simulink model "AMCLIB_SpeedLoop_BAM"  (Simulink 9.3)
settings: Solver=VariableStepAuto  StartTime=0.0  StopTime=10.0  RelTol=1e-3
settings Model: Creator=nxa18952  LastModifiedBy=nxa18952
settings DataIOCC: SaveFormat=Dataset  SignalLoggingSaveFormat=Dataset  ReturnWorkspaceOutputs=on
settings OptimizationCC: LifeSpan=auto
settings DebuggingCC: UnderspecifiedInitializationDetection=Simplified  MergeDetectMultiDrivingBlocksExec=error  FcnCallInpInsideContextMsg=error  SFUnexpectedBacktrackingDiag=error  SFNoUnconditionalDefaultTransitionDiag=error  SFExecutionAtInitializationDiag=warning  ArithmeticOperatorsInVariantConditions=error
settings HardwareCC: ProdBitPerPointer=64  ProdBitPerSizeT=64  ProdBitPerPtrDiffT=64  ProdLargestAtomicFloat=Float  ProdIntDivRoundTo=Zero  ProdEndianess=LittleEndian  ProdWordSize=64  ProdHWDeviceType=Intel->x86-64 (Windows64)
settings ModelReferenceCC: PropagateSignalLabelsOutOfModel=on
settings SFSimCC: SimUseLocalCustomCode=on
settings RTWCC: RTWUseLocalCustomCode=on
settings CodeAppCC: StateflowObjectComments=off
settings GRTTargetCC: TargetLangStandard=C99 (ISO)  CombineOutputUpdateFcns=on  GRTInterface=off
settings ConfigComp: CovMetricSettings=dwe  CovHtmlReporting=off  CovSaveCumulativeToWorkspaceVar=off  CovSaveSingleToWorkspaceVar=off  CovExternalEMLEnable=on

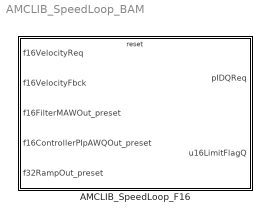
== system AMCLIB_SpeedLoop_BAM ==
  AMCLIB_SpeedLoop_F16 : Subsystem  TreatAsAtomicUnit=on  mask(AMCLIB_SpeedLoop_F16){showStates=Hide (faster execution), resetStatesEnable=Pre-set according to the first set of inputs after reset, showDebugOutputs=Hide, u16NSamplesW=0, f16PropGainQ=0, f16IntegGainQ=0, s16PropGainShiftQ=0, s16IntegGainShiftQ=0, f16LowerLimitQ=0, f16UpperLimitQ=0, f32RampUp=0, f32RampDown=0}
      mask prompts: showStates "Show internal states"; resetStatesEnable "Internal state after reset"; showDebugOutputs "Show debugging outputs"; u16NSamplesW "u16NSamplesW (GDFLIB_FilterMA - recalculated smoothing factor)"; f16PropGainQ "f16PropGainQ (GFLIB_ControllerPIpAW - proportional gain)"; f16IntegGainQ "f16IntegGainQ (GFLIB_ControllerPIpAW - integral gain)"; s16PropGainShiftQ "s16PropGainShiftQ (GFLIB_ControllerPIpAW - scaling bitwise shift applied to the proportional gain)"; s16IntegGainShiftQ "s16IntegGainShiftQ (GFLIB_ControllerPIpAW - scaling bitwise shift applied to the integral gain)"; f16LowerLimitQ "f16LowerLimitQ (GFLIB_ControllerPIpAW - lower limit)"; f16UpperLimitQ "f16UpperLimitQ (GFLIB_ControllerPIpAW - upper limit)"; f32RampUp "f32RampUp (Ramp up increment coefficient)"; f32RampDown "f32RampDown (Ramp decrement coefficient)"
      mask help: Speed loop controller for the PMSM field-oriented control algorithm in 16-bit fixed-point fractional implementation. This block supports re-initialization of the internal state during simulation. If the block is reset, the outputs of the MA filter, PI controller, and the ramp will be aligned with the inputs f16FilterMAWOut_preset, f16ControllerPIpAWQOut_preset, and f32RampOut_preset. Refer to the AMMCLIB User's Guide for further details.
      mask init:
      | if ~evalin('base','exist(''tS8'',''var'')')
      |   if (2 ~= exist('SWLIBS_Typedefs.mat','file'))
      |       error('File SWLIBS_Typedefs.mat is not on the Matlab path. Please add the AMMCLIB "bam" folder in the Matlab Search Path.');
      |   else
      |       evalin('base', 'load(''SWLIBS_Typedefs.mat'')');
      |   end
      | end
      | if showStates == 1
      |     % hidden state variables
      |     if strcmp(get_param([gcb '/u16NSamplesW'], 'BlockType'), 'Inport')
      |         posblk = get_param(gcb, 'Position');
      | 
      |         pos = get_param(    [gcb, '/u16NSamplesW'], 'Position');
      |         orient = get_param( [gcb, '/u16NSamplesW'], 'Orientation');
      |         delete_block(       [gcb, '/u16NSamplesW']);
      |         add_block('built-in/Ground', [gcb, '/u16NSamplesW'], 'Position', pos, 'Orientation', orient);
      | 
      |         pos = get_param(    [gcb, '/f16PropGainQ'], 'Position');
      |         orient = get_param( [gcb, '/f16PropGainQ'], 'Orientation');
      |         delete_block(       [gcb, '/f16PropGainQ']);
      |         add_block('built-in/Ground', [gcb, '/f16PropGainQ'], 'Position', pos, 'Orientation', orient);
      | 
      |         pos = get_param(    [gcb, '/f16IntegGainQ'], 'Position');
      |         orient = get_param( [gcb, '/f16IntegGainQ'], 'Orientation');
      |         delete_block(       [gcb, '/f16IntegGainQ']);
      |         add_block('built-in/Ground', [gcb, '/f16IntegGainQ'], 'Position', pos, 'Orientation', orient);
      | 
      |         pos = get_param(    [gcb, '/s16PropGainShiftQ'], 'Position');
      |         orient = get_param( [gcb, '/s16PropGainShiftQ'], 'Orientation');
      |         delete_block(       [gcb, '/s16PropGainShiftQ']);
      |         add_block('built-in/Ground', [gcb, '/s16PropGainShiftQ'], 'Position', pos, 'Orientation', orient);
      | 
      |         pos = get_param(    [gcb, '/s16IntegGainShiftQ'], 'Position');
      |         orient = get_param( [gcb, '/s16IntegGainShiftQ'], 'Orientation');
      |         delete_block(       [gcb, '/s16IntegGainShiftQ']);
      |         add_block('built-in/Ground', [gcb, '/s16IntegGainShiftQ'], 'Position', pos, 'Orientation', orient);
      | 
      |         pos = get_param(    [gcb, '/f16LowerLimitQ'], 'Position');
      |         orient = get_param( [gcb, '/f16LowerLimitQ'], 'Orientation');
      |         delete_block(       [gcb, '/f16LowerLimitQ']);
      |         add_block('built-in/Ground', [gcb, '/f16LowerLimitQ'], 'Position', pos, 'Orientation', orient);
      | 
      |         pos = get_param(    [gcb, '/f16UpperLimitQ'], 'Position');
      |         orient = get_param( [gcb, '/f16UpperLimitQ'], 'Orientation');
      |         delete_block(       [gcb, '/f16UpperLimitQ']);
      |         add_block('built-in/Ground', [gcb, '/f16UpperLimitQ'], 'Position', pos, 'Orientation', orient);
      | 
      |         pos = get_param(    [gcb, '/f32RampUp'], 'Position');
      |         orient = get_param( [gcb, '/f32RampUp'], 'Orientation');
      |         delete_block(       [gcb, '/f32RampUp']);
      |         add_block('built-in/Ground', [gcb, '/f32RampUp'], 'Position', pos, 'Orientation', orient);
      | 
      |         pos = get_param(    [gcb, '/f32RampDown'], 'Position');
      |         orient = get_param( [gcb, '/f32RampDown'], 'Orientation');
      |         delete_block(       [gcb, '/f32RampDown']);
      |         add_block('built-in/Ground', [gcb, '/f32RampDown'], 'Position', pos, 'Orientation', orient);
      | 
      |         pos = get_param(    [gcb, '/f32AccW'], 'Position');
      |         orient = get_param( [gcb, '/f32AccW'], 'Orientation');
      |         delete_block(       [gcb, '/f32AccW']);
      |         add_block('built-in/Ground', [gcb, '/f32AccW'], 'Position', pos, 'Orientation', orient);
      | 
      |         pos = get_param(    [gcb, '/f32IntegPartK_1Q'], 'Position');
      |         orient = get_param( [gcb, '/f32IntegPartK_1Q'], 'Orientation');
      |         delete_block(       [gcb, '/f32IntegPartK_1Q']);
      |         add_block('built-in/Ground', [gcb, '/f32IntegPartK_1Q'], 'Position', pos, 'Orientation', orient);
      | 
      |         pos = get_param(    [gcb, '/f16InK_1Q'], 'Position');
      |         orient = get_param( [gcb, '/f16InK_1Q'], 'Orientation');
      |         delete_block(       [gcb, '/f16InK_1Q']);
      |         add_block('built-in/Ground', [gcb, '/f16InK_1Q'], 'Position', pos, 'Orientation', orient);
      | 
      |         pos = get_param(    [gcb, '/f32State'], 'Position');
      |         orient = get_param( [gcb, '/f32State'], 'Orientation');
      |         delete_block(       [gcb, '/f32State']);
      |         add_block('built-in/Ground', [gcb, '/f32State'], 'Position', pos, 'Orientation', orient);
      | 
      | 
      |         pos = get_param(    [gcb '/f32AccW_Out'], 'Position');
      |         orient = get_param( [gcb '/f32AccW_Out'], 'Orientation');
      |         delete_block(       [gcb '/f32AccW_Out']);
      |         add_block('built-in/Terminator', [gcb '/f32AccW_Out'], 'Position', pos, 'Orientation', orient);
      | 
      |         pos = get_param(    [gcb '/f32IntegPartK_1Q_Out'], 'Position');
      |         orient = get_param( [gcb '/f32IntegPartK_1Q_Out'], 'Orientation');
      |         delete_block(       [gcb '/f32IntegPartK_1Q_Out']);
      |         add_block('built-in/Terminator', [gcb '/f32IntegPartK_1Q_Out'], 'Position', pos, 'Orientation', orient);
      | 
      |         pos = get_param(    [gcb '/f16InK_1Q_Out'], 'Position');
      |         orient = get_param( [gcb '/f16InK_1Q_Out'], 'Orientation');
      |         delete_block(       [gcb '/f16InK_1Q_Out']);
      |         add_block('built-in/Terminator', [gcb '/f16InK_1Q_Out'], 'Position', pos, 'Orientation', orient);
      | 
      |         pos = get_param(    [gcb '/f32State_Out'], 'Position');
      |         orient = get_param( [gcb '/f32State_Out'], 'Orientation');
      |         delete_block(       [gcb '/f32State_Out']);
      |         add_block('built-in/Terminator', [gcb '/f32State_Out'], 'Position', pos, 'Orientation', orient);
      | 
      | 
      |         if strcmp(get_param([gcb '/f16WReqFilt'], 'BlockType'), 'Outport')
      |             pos = get_param(    [gcb '/f16WReqFilt'], 'Position');
      |             orient = get_param( [gcb '/f16WReqFilt'], 'Orientation');
      |             delete_block(       [gcb '/f16WReqFilt']);
      |             add_block('built-in/Terminator', [gcb '/f16WReqFilt'], 'Position', pos, 'Orientation', orient);
      | 
      |             pos = get_param(    [gcb '/f16WErr'], 'Position');
      |             orient = get_param( [gcb '/f16WErr'], 'Orientation');
      |             delete_block(       [gcb '/f16WErr']);
      |             add_block('built-in/Terminator', [gcb '/f16WErr'], 'Position', pos, 'Orientation', orient);
      | 
      |             pos = get_param(    [gcb '/f16WFbckFilt'], 'Position');
      |             orient = get_param( [gcb '/f16WFbckFilt'], 'Orientation');
      |             delete_block(       [gcb '/f16WFbckFilt']);
      |             add_block('built-in/Terminator', [gcb '/f16WFbckFilt'], 'Position', pos, 'Orientation', orient);
      | 
      |         end
      | 
      |         set_param([gcb '/f16VelocityReq'], 'Port', '1');
      |         set_param([gcb '/f16VelocityFbck'], 'Port', '2');
      |         set_param([gcb '/f16FilterMAWOut_preset'], 'Port', '3');
      |         set_param([gcb '/f16ControllerPIpAWQOut_preset'], 'Port', '4');
      |         set_param([gcb '/f32RampOut_preset'], 'Port', '5');
      | 
      |         set_param([gcb '/pIDQReq'], 'Port', '1');
      |         set_param([gcb '/u16LimitFlagQ'], 'Port', '2');
      | 
      |         set_param(gcb,'MaskEnables',{'on','on','off','on','on','on','on','on','on','on','on','on'});
      | 
      |         if (posblk(4) - posblk(2)) > 150
      |           height = 150;
      |           set_param(gcb,'Position',[posblk(1), posblk(2), posblk(3), posblk(2)+height])
      |         end
      |     end
      | else
      |     % shown state variables
      |     if strcmp(get_param([gcb '/u16NSamplesW'], 'BlockType'), 'Ground')
      |         posblk = get_param(gcb, 'Position');
      | 
      |         pos = get_param(    [gcb, '/u16NSamplesW'], 'Position');
      |         orient = get_param( [gcb, '/u16NSamplesW'], 'Orientation');
      |         delete_block(       [gcb, '/u16NSamplesW']);
      |         add_block('built-in/Inport', [gcb, '/u16NSamplesW'], 'Position', pos, 'Orientation', orient, 'OutDataTypeStr', 'uint16');
      | 
      |         pos = get_param(    [gcb, '/f16PropGainQ'], 'Position');
      |         orient = get_param( [gcb, '/f16PropGainQ'], 'Orientation');
      |         delete_block(       [gcb, '/f16PropGainQ']);
      |         add_block('built-in/Inport', [gcb, '/f16PropGainQ'], 'Position', pos, 'Orientation', orient, 'OutDataTypeStr', 'int16');
      | 
      |         pos = get_param(    [gcb, '/f16IntegGainQ'], 'Position');
      |         orient = get_param( [gcb, '/f16IntegGainQ'], 'Orientation');
      |         delete_block(       [gcb, '/f16IntegGainQ']);
      |         add_block('built-in/Inport', [gcb, '/f16IntegGainQ'], 'Position', pos, 'Orientation', orient, 'OutDataTypeStr', 'int16');
      | 
      |         pos = get_param(    [gcb, '/s16PropGainShiftQ'], 'Position');
      |         orient = get_param( [gcb, '/s16PropGainShiftQ'], 'Orientation');
      |         delete_block(       [gcb, '/s16PropGainShiftQ']);
      |         add_block('built-in/Inport', [gcb, '/s16PropGainShiftQ'], 'Position', pos, 'Orientation', orient, 'OutDataTypeStr', 'int16');
      | 
      |         pos = get_param(    [gcb, '/s16IntegGainShiftQ'], 'Position');
      |         orient = get_param( [gcb, '/s16IntegGainShiftQ'], 'Orientation');
      |         delete_block(       [gcb, '/s16IntegGainShiftQ']);
      |         add_block('built-in/Inport', [gcb, '/s16IntegGainShiftQ'], 'Position', pos, 'Orientation', orient, 'OutDataTypeStr', 'int16');
      | 
      |         pos = get_param(    [gcb, '/f16LowerLimitQ'], 'Position');
      |         orient = get_param( [gcb, '/f16LowerLimitQ'], 'Orientation');
      |         delete_block(       [gcb, '/f16LowerLimitQ']);
      |         add_block('built-in/Inport', [gcb, '/f16LowerLimitQ'], 'Position', pos, 'Orientation', orient, 'OutDataTypeStr', 'int16');
      | 
      |         pos = get_param(    [gcb, '/f16UpperLimitQ'], 'Position');
      |         orient = get_param( [gcb, '/f16UpperLimitQ'], 'Orientation');
      |         delete_block(       [gcb, '/f16UpperLimitQ']);
      |         add_block('built-in/Inport', [gcb, '/f16UpperLimitQ'], 'Position', pos, 'Orientation', orient, 'OutDataTypeStr', 'int16');
      | 
      |         pos = get_param(    [gcb, '/f32RampUp'], 'Position');
      |         orient = get_param( [gcb, '/f32RampUp'], 'Orientation');
      |         delete_block(       [gcb, '/f32RampUp']);
      |         add_block('built-in/Inport', [gcb, '/f32RampUp'], 'Position', pos, 'Orientation', orient, 'OutDataTypeStr', 'int32');
      | 
      |         pos = get_param(    [gcb, '/f32RampDown'], 'Position');
      |         orient = get_param( [gcb, '/f32RampDown'], 'Orientation');
      |         delete_block(       [gcb, '/f32RampDown']);
      |         add_block('built-in/Inport', [gcb, '/f32RampDown'], 'Position', pos, 'Orientation', orient, 'OutDataTypeStr', 'int32');
      | 
      |         pos = get_param(    [gcb, '/f32AccW'], 'Position');
      |         orient = get_param( [gcb, '/f32AccW'], 'Orientation');
      |         delete_block(       [gcb, '/f32AccW']);
      |         add_block('built-in/Inport', [gcb, '/f32AccW'], 'Position', pos, 'Orientation', orient, 'OutDataTypeStr', 'int32');
      | 
      |         pos = get_param(    [gcb, '/f32IntegPartK_1Q'], 'Position');
      |         orient = get_param( [gcb, '/f32IntegPartK_1Q'], 'Orientation');
      |         delete_block(       [gcb, '/f32IntegPartK_1Q']);
      |         add_block('built-in/Inport', [gcb, '/f32IntegPartK_1Q'], 'Position', pos, 'Orientation', orient, 'OutDataTypeStr', 'int32');
      | 
      |         pos = get_param(    [gcb, '/f16InK_1Q'], 'Position');
      |         orient = get_param( [gcb, '/f16InK_1Q'], 'Orientation');
      |         delete_block(       [gcb, '/f16InK_1Q']);
      |         add_block('built-in/Inport', [gcb, '/f16InK_1Q'], 'Position', pos, 'Orientation', orient, 'OutDataTypeStr', 'int16');
      | 
      |         pos = get_param(    [gcb, '/f32State'], 'Position');
      |         orient = get_param( [gcb, '/f32State'], 'Orientation');
      |         delete_block(       [gcb, '/f32State']);
      |         add_block('built-in/Inport', [gcb, '/f32State'], 'Position', pos, 'Orientation', orient, 'OutDataTypeStr', 'int32');
      | 
      | 
      |         pos = get_param(    [gcb '/f32AccW_Out'], 'Position');
      |         orient = get_param( [gcb '/f32AccW_Out'], 'Orientation');
      |         delete_block(       [gcb '/f32AccW_Out']);
      |         add_block('built-in/Outport', [gcb '/f32AccW_Out'], 'Position', pos, 'Orientation', orient);
      | 
      |         pos = get_param(    [gcb '/f32IntegPartK_1Q_Out'], 'Position');
      |         orient = get_param( [gcb '/f32IntegPartK_1Q_Out'], 'Orientation');
      |         delete_block(       [gcb '/f32IntegPartK_1Q_Out']);
      |         add_block('built-in/Outport', [gcb '/f32IntegPartK_1Q_Out'], 'Position', pos, 'Orientation', orient);
      | 
      |         pos = get_param(    [gcb '/f16InK_1Q_Out'], 'Position');
      |         orient = get_param( [gcb '/f16InK_1Q_Out'], 'Orientation');
      |         delete_block(       [gcb '/f16InK_1Q_Out']);
      |         add_block('built-in/Outport', [gcb '/f16InK_1Q_Out'], 'Position', pos, 'Orientation', orient);
      | 
      |         pos = get_param(    [gcb '/f32State_Out'], 'Position');
      |         orient = get_param( [gcb '/f32State_Out'], 'Orientation');
      |         delete_block(       [gcb '/f32State_Out']);
      |         add_block('built-in/Outport', [gcb '/f32State_Out'], 'Position', pos, 'Orientation', orient);
      | 
      | 
      |         if (showDebugOutputs == 2) && (strcmp(get_param([gcb '/f16WReqFilt'], 'BlockType'), 'Terminator'))
      |             pos = get_param(    [gcb '/f16WReqFilt'], 'Position');
      |             orient = get_param( [gcb '/f16WReqFilt'], 'Orientation');
      |             delete_block(       [gcb '/f16WReqFilt']);
      |             add_block('built-in/Outport', [gcb '/f16WReqFilt'], 'Position', pos, 'Orientation', orient);
      | 
      |             pos = get_param(    [gcb '/f16WErr'], 'Position');
      |             orient = get_param( [gcb '/f16WErr'], 'Orientation');
      |             delete_block(       [gcb '/f16WErr']);
      |             add_block('built-in/Outport', [gcb '/f16WErr'], 'Position', pos, 'Orientation', orient);
      | 
      |             pos = get_param(    [gcb '/f16WFbckFilt'], 'Position');
      |             orient = get_param( [gcb '/f16WFbckFilt'], 'Orientation');
      |             delete_block(       [gcb '/f16WFbckFilt']);
      |             add_block('built-in/Outport', [gcb '/f16WFbckFilt'], 'Position', pos, 'Orientation', orient);
      | 
      |         end
      | 
      |         set_param([gcb '/f16VelocityReq'], 'Port', '1');
      |         set_param([gcb '/f16VelocityFbck'], 'Port', '2');
      |         set_param([gcb '/f16FilterMAWOut_preset'], 'Port', '3');
      |         set_param([gcb '/f16ControllerPIpAWQOut_preset'], 'Port', '4');
      |         set_param([gcb '/f32RampOut_preset'], 'Port', '5');
      |         set_param([gcb '/u16NSamplesW'], 'Port', '6');
      |         set_param([gcb '/f16PropGainQ'], 'Port', '7');
      |         set_param([gcb '/f16IntegGainQ'], 'Port', '8');
      |         set_param([gcb '/s16PropGainShiftQ'], 'Port', '9');
      |         set_param([gcb '/s16IntegGainShiftQ'], 'Port', '10');
      |         set_param([gcb '/f16LowerLimitQ'], 'Port', '11');
      |         set_param([gcb '/f16UpperLimitQ'], 'Port', '12');
      |         set_param([gcb '/f32RampUp'], 'Port', '13');
      |         set_param([gcb '/f32RampDown'], 'Port', '14');
      |         set_param([gcb '/f32AccW'], 'Port', '15');
      |         set_param([gcb '/f32IntegPartK_1Q'], 'Port', '16');
      |         set_param([gcb '/f16InK_1Q'], 'Port', '17');
      |         set_param([gcb '/f32State'], 'Port', '18');
      | 
      |         if (showDebugOutputs == 2)
      |             set_param([gcb '/pIDQReq'], 'Port', '1');
      |             set_param([gcb '/u16LimitFlagQ'], 'Port', '2');
      |             set_param([gcb '/f16WReqFilt'], 'Port', '3');
      |             set_param([gcb '/f16WErr'], 'Port', '4');
      |             set_param([gcb '/f16WFbckFilt'], 'Port', '5');
      |             set_param([gcb '/f32AccW_Out'], 'Port', '6');
      |             set_param([gcb '/f32IntegPartK_1Q_Out'], 'Port', '7');
      |             set_param([gcb '/f16InK_1Q_Out'], 'Port', '8');
      |             set_param([gcb '/f32State_Out'], 'Port', '9');
      |         else
      |             set_param([gcb '/pIDQReq'], 'Port', '1');
      |             set_param([gcb '/u16LimitFlagQ'], 'Port', '2');
      |             set_param([gcb '/f32AccW_Out'], 'Port', '3');
      |             set_param([gcb '/f32IntegPartK_1Q_Out'], 'Port', '4');
      |             set_param([gcb '/f16InK_1Q_Out'], 'Port', '5');
      |             set_param([gcb '/f32State_Out'], 'Port', '6');
      |         end
      | 
      |         set_param(gcb,'MaskEnables',{'on','on','on','off','off','off','off','off','off','off','off','off'});
      | 
      |         if (posblk(4) - posblk(2)) < 475
      |           height = 475;
      |           set_param(gcb,'Position',[posblk(1), posblk(2), posblk(3), posblk(2)+height])
      |         end
      |     else
      |         if (showDebugOutputs == 2) && (strcmp(get_param([gcb '/f16WReqFilt'], 'BlockType'), 'Terminator'))
      |             % shown debugging outputs
      |             pos = get_param(    [gcb '/f16WReqFilt'], 'Position');
      |             orient = get_param( [gcb '/f16WReqFilt'], 'Orientation');
      |             delete_block(       [gcb '/f16WReqFilt']);
      |             add_block('built-in/Outport', [gcb '/f16WReqFilt'], 'Position', pos, 'Orientation', orient);
      | 
      |             pos = get_param(    [gcb '/f16WErr'], 'Position');
      |             orient = get_param( [gcb '/f16WErr'], 'Orientation');
      |             delete_block(       [gcb '/f16WErr']);
      |             add_block('built-in/Outport', [gcb '/f16WErr'], 'Position', pos, 'Orientation', orient);
      | 
      |             pos = get_param(    [gcb '/f16WFbckFilt'], 'Position');
      |             orient = get_param( [gcb '/f16WFbckFilt'], 'Orientation');
      |             delete_block(       [gcb '/f16WFbckFilt']);
      |             add_block('built-in/Outport', [gcb '/f16WFbckFilt'], 'Position', pos, 'Orientation', orient);
      | 
      |             set_param([gcb '/pIDQReq'], 'Port', '1');
      |             set_param([gcb '/u16LimitFlagQ'], 'Port', '2');
      |             set_param([gcb '/f16WReqFilt'], 'Port', '3');
      |             set_param([gcb '/f16WErr'], 'Port', '4');
      |             set_param([gcb '/f16WFbckFilt'], 'Port', '5');
      |             set_param([gcb '/f32AccW_Out'], 'Port', '6');
      |             set_param([gcb '/f32IntegPartK_1Q_Out'], 'Port', '7');
      |             set_param([gcb '/f16InK_1Q_Out'], 'Port', '8');
      |             set_param([gcb '/f32State_Out'], 'Port', '9');
      |         elseif (showDebugOutputs == 1) && (strcmp(get_param([gcb '/f16WReqFilt'], 'BlockType'), 'Outport'))
      |             % hidden debugging outputs
      |             pos = get_param(    [gcb '/f16WReqFilt'], 'Position');
      |             orient = get_param( [gcb '/f16WReqFilt'], 'Orientation');
      |             delete_block(       [gcb '/f16WReqFilt']);
      |             add_block('built-in/Terminator', [gcb '/f16WReqFilt'], 'Position', pos, 'Orientation', orient);
      | 
      |             pos = get_param(    [gcb '/f16WErr'], 'Position');
      |             orient = get_param( [gcb '/f16WErr'], 'Orientation');
      |             delete_block(       [gcb '/f16WErr']);
      |             add_block('built-in/Terminator', [gcb '/f16WErr'], 'Position', pos, 'Orientation', orient);
      | 
      |             pos = get_param(    [gcb '/f16WFbckFilt'], 'Position');
      |             orient = get_param( [gcb '/f16WFbckFilt'], 'Orientation');
      |             delete_block(       [gcb '/f16WFbckFilt']);
      |             add_block('built-in/Terminator', [gcb '/f16WFbckFilt'], 'Position', pos, 'Orientation', orient);
      | 
      |             set_param([gcb '/pIDQReq'], 'Port', '1');
      |             set_param([gcb '/u16LimitFlagQ'], 'Port', '2');
      |             set_param([gcb '/f32AccW_Out'], 'Port', '3');
      |             set_param([gcb '/f32IntegPartK_1Q_Out'], 'Port', '4');
      |             set_param([gcb '/f16InK_1Q_Out'], 'Port', '5');
      |             set_param([gcb '/f32State_Out'], 'Port', '6');
      |         end
      |     end
      | end
      settings: RTWSystemCode=Inline
      mask TypeOptions showStates: Hide (faster execution) | Show (allows debugging; connect feedback loops manually)
      mask Callback showStates:
      | maskStr = get_param(gcb,'showStates');
      | if strcmp(maskStr,'Hide (faster execution)'),
      |     set_param(gcb,'MaskEnables',{'on','on','off','on','on','on','on','on','on','on','on','on'});
      | else
      |     set_param(gcb,'MaskEnables',{'on','on','on','off','off','off','off','off','off','off','off','off'});
      | end
      mask TypeOptions resetStatesEnable: Pre-set according to the first set of inputs after reset | Clear to zero
      mask TypeOptions showDebugOutputs: Hide | Show
      mask Display:
      | color('black');
      | pos = get_param(gcb, 'Position');
      | width = pos(3) - pos(1);
      | height = pos(4) - pos(2);
      | tX=width/2;
      | tY=height - 25;
      | color('black');
      | text(tX,tY, 'AMCLIB_SpeedLoop_F16', 'horizontalAlignment', 'center');
      | if showStates == 2
      |   color('red');
      |   text(tX,tY - 20, ['debugging mode' char(13) char(10) '(limited performance)'], 'horizontalAlignment', 'center');
      | end

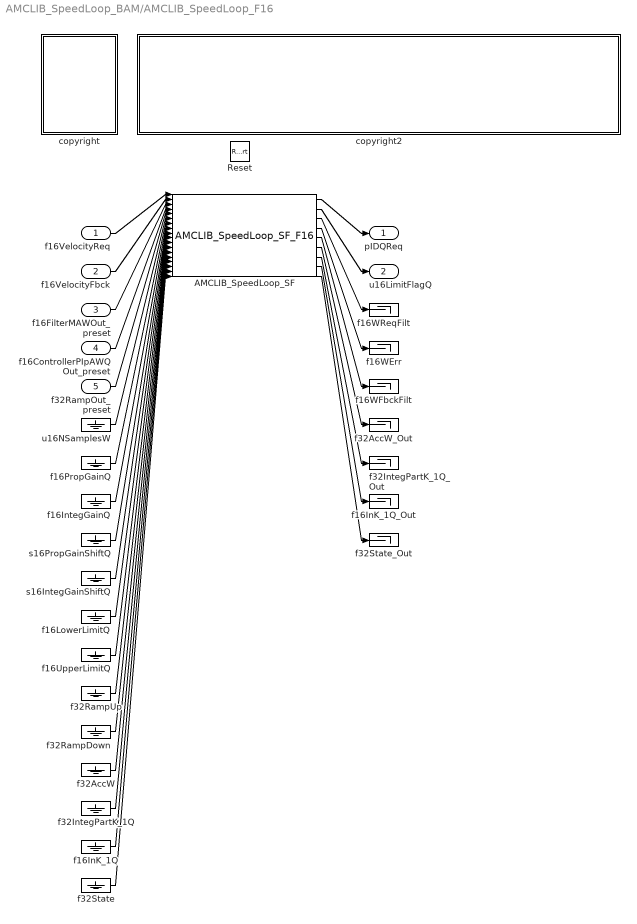
== system AMCLIB_SpeedLoop_BAM/AMCLIB_SpeedLoop_F16 ==
  f16VelocityReq : Inport  OutDataTypeStr=int16
  f16VelocityFbck : Inport  Port=2  OutDataTypeStr=int16
  f16FilterMAWOut_preset : Inport  Port=3  OutDataTypeStr=int16
  f16ControllerPIpAWQOut_preset : Inport  Port=4  OutDataTypeStr=int16
  f32RampOut_preset : Inport  Port=5  OutDataTypeStr=int32
  Reset : ResetPort  DisableCoverage=on
  AMCLIB_SpeedLoop_SF : S-Function  FunctionName=AMCLIB_SpeedLoop_SF_F16  Parameters=showStates,resetStatesEnable,showDebugOutputs,u16NSamplesW,f16PropGainQ,f16IntegGainQ,s16PropGainShiftQ,s16IntegGainShiftQ,f16LowerLimitQ,f16UpperLimitQ,f32RampUp,f32RampDown  SFunctionDeploymentMode=off  EnableBusSupport=off
  copyright : Subsystem
      mask Display: text(10,90,'FILE:');text(10,75,'DESRIPTION:');text(10,60,'COPYRIGHT:');text(10,45,'VERSION:');text(10,30,'DATE:')
  copyright2 : Subsystem
      mask Display: text(10,90,'AMCLIB_SpeedLoop_BAM_F16.mdl');text(10,75,'PMSM Speed Loop Controller.');text(10,60,'NXP 2020');text(10,45,'1.0');text(10,30,'28-Mar-2020');
  f16InK_1Q : Ground
  f16InK_1Q_Out : Terminator
  f16IntegGainQ : Ground
  f16LowerLimitQ : Ground
  f16PropGainQ : Ground
  f16UpperLimitQ : Ground
  f16WErr : Terminator
  f16WFbckFilt : Terminator
  f16WReqFilt : Terminator
  f32AccW : Ground
  f32AccW_Out : Terminator
  f32IntegPartK_1Q : Ground
  f32IntegPartK_1Q_Out : Terminator
  f32RampDown : Ground
  f32RampUp : Ground
  f32State : Ground
  f32State_Out : Terminator
  s16IntegGainShiftQ : Ground
  s16PropGainShiftQ : Ground
  u16NSamplesW : Ground
  pIDQReq : Outport
  u16LimitFlagQ : Outport  Port=2
  wires:
  f16VelocityReq/1 -> AMCLIB_SpeedLoop_SF/1
  f16VelocityFbck/1 -> AMCLIB_SpeedLoop_SF/2
  f16FilterMAWOut_preset/1 -> AMCLIB_SpeedLoop_SF/3
  f16ControllerPIpAWQOut_preset/1 -> AMCLIB_SpeedLoop_SF/4
  f32RampOut_preset/1 -> AMCLIB_SpeedLoop_SF/5
  u16NSamplesW/1 -> AMCLIB_SpeedLoop_SF/6
  f16PropGainQ/1 -> AMCLIB_SpeedLoop_SF/7
  f16IntegGainQ/1 -> AMCLIB_SpeedLoop_SF/8
  s16PropGainShiftQ/1 -> AMCLIB_SpeedLoop_SF/9
  s16IntegGainShiftQ/1 -> AMCLIB_SpeedLoop_SF/10
  f16LowerLimitQ/1 -> AMCLIB_SpeedLoop_SF/11
  f16UpperLimitQ/1 -> AMCLIB_SpeedLoop_SF/12
  f32RampUp/1 -> AMCLIB_SpeedLoop_SF/13
  f32RampDown/1 -> AMCLIB_SpeedLoop_SF/14
  f32AccW/1 -> AMCLIB_SpeedLoop_SF/15
  f32IntegPartK_1Q/1 -> AMCLIB_SpeedLoop_SF/16
  f16InK_1Q/1 -> AMCLIB_SpeedLoop_SF/17
  f32State/1 -> AMCLIB_SpeedLoop_SF/18
  AMCLIB_SpeedLoop_SF/1 -> pIDQReq/1
  AMCLIB_SpeedLoop_SF/2 -> u16LimitFlagQ/1
  AMCLIB_SpeedLoop_SF/3 -> f16WReqFilt/1
  AMCLIB_SpeedLoop_SF/4 -> f16WErr/1
  AMCLIB_SpeedLoop_SF/5 -> f16WFbckFilt/1
  AMCLIB_SpeedLoop_SF/6 -> f32AccW_Out/1
  AMCLIB_SpeedLoop_SF/7 -> f32IntegPartK_1Q_Out/1
  AMCLIB_SpeedLoop_SF/8 -> f16InK_1Q_Out/1
  AMCLIB_SpeedLoop_SF/9 -> f32State_Out/1

== system AMCLIB_SpeedLoop_BAM/AMCLIB_SpeedLoop_F16/copyright ==

== system AMCLIB_SpeedLoop_BAM/AMCLIB_SpeedLoop_F16/copyright2 ==
